simulink model "amplificator_function"  (R2022b)
settings: Solver=VariableStepAuto  StartTime=0.0  StopTime=10.0  RelTol=1e-3
settings Model: Creator=Ruxandra  LastModifiedBy=Ruxandra

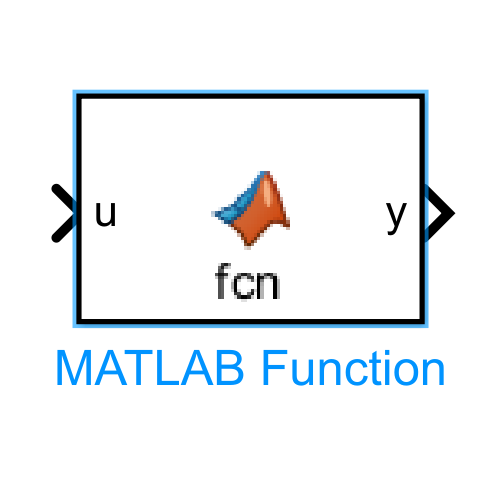
[thumbnail: Simulink's stored preview of the top-level diagram]
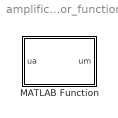
== system amplificator_function ==
  MATLAB Function : MATLAB Function  TreatAsAtomicUnit=on

== matlab function amplificator_function/MATLAB Function ==
  data: ua input; um output
function um = amp(ua)
um=2.2*ua;
if um<0; um=0; end
if ua>8.1; um = um+5*(ua-8.1); end
if um>22; um=22; end
